simulink library "X8_lib"  (R2015a)
settings: Solver=ode45  StartTime=0.0  StopTime=10.0  RelTol=1e-3
values from neighbouring files (symbols this model uses):
  P = computeGains(T_phi_delta_a,T_v_delta_r,T_theta_delta_e,T_Va_theta,T_Va_delta_t,P)    [initX8_demo.m]
  T_elevon2ailelev = [1 1 ... (first row only)    [init.m]
  x0 = [eta_0', ny_0' zeros(1,6)]'    [init.m]    (also in runX8.m = [-0.0000    0.0000 -100.0000   0.9997    0.0000    0.0232   ; trimX8.m = [0 0 -h_ini         quat0(1) quat0(2) quat0(3)   quat0(4)   )
undefined symbols (not defined in the file or in its folder): F, Light, MIL
libraries: aerolibactuator x6, aerolibutil x2, aerolibwind2 x2, aerolibtransform2 x1
settings Model: Creator=krisgry  LastModifiedBy=krisgry

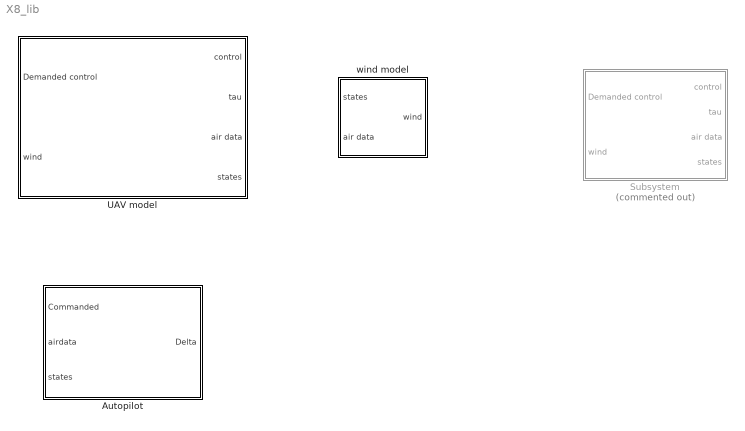
== system X8_lib ==
  Autopilot : Subsystem  mask{param='x8_param', X_trim=[0.0000    0.0000 -150.0000    0.9997    0.0000    0.0232   -0.0000 18.0168    0.0001    0.8366    0.0000    0.0000    0.0000 0.0039 -0.0000    0.0039   -0.0000    0.1240]', U_trim=[0.0079    0.0000         0    0.1240]'}
      mask prompts: param "UAV model"
      mask help:
      | UAV model can be either 'x8_param' or 'aerosonde'
      |
      | # Inputs:
      | Commanded: a 3x1 vector consisting of desired [airspeed, height, course angle]
      | airdata: a 10-element bus with airspeed, alpha, beta ... see bus_definitions.m
      | states: a bus consisting of 6 buses: position, attitude, quaternion, velocity, angular velocity, acceleration. See bus_definitions.m
      |
      | # Outputs:
      | delta: the control vector calculated by the autopilot
      mask init:
      | if(~exist('P') || ~isfield(P,'course_ki'))
      |     init;
      |     P.tau = 1; %Time constant for the band-limited differentiator
      |     P.u_trim = U_trim;
      |     [T_phi_delta_a,T_chi_phi,T_theta_delta_e,T_h_theta,T_h_Va,T_Va_delta_t,T_Va_theta,T_v_delta_r]= compute_tf_model(X_trim,U_trim,P);
      |     P=computeGains(T_phi_delta_a,T_v_delta_r,T_theta_delta_e,T_Va_theta,T_Va_delta_t,P);
      |    [phi0,theta0,psi0] = q2euler(X_trim(4:7)/norm(X_trim(4:7))); 
      | end
  Subsystem : Subsystem  Commented=on  mask{param='x8_param', pos0=[0 0 0], quat0=[1,0,0,0], vel0=[0 0 0], rate0=[0,0,0], servoR_pos0=0, servoR_vel0=0, servoL_pos0=0, servoL_vel0=0, prop_speed0=0}
      mask prompts: param "UAV model"; pos0 "NED position"; quat0 "Quaternion"; vel0 "Velocity"; rate0 "Angular velocity"; servoR_pos0 "Right servo deflection"; servoR_vel0 "Right servo deflection"; servoL_pos0 "Left servo deflection"; servoL_vel0 "Left servo speed"; prop_speed0 "Motor speed"
      mask help:
      | UAV model can be either 'x8_param' or 'aerosonde'
      |
      | #### Inputs:
      | Demanded control: a 4x1 vector consisting of [elevator, aileron, rudder, throttle]
      | wind: a 6x1 vector consisting of the wind+gust in NED, and the body rate gusts: [N,E,D,p,q,r]
      |
      | #### Outputs:
      | control: the control vector after it has been passed through the actuator model
      | tau: a 6x1 force/moment vector: [Fx,Fy,Fz,l,m,n]
      | airdata: a 10-element bus with airspeed, alpha, beta ... see bus_definitions.m
      | states: a bus consisting of 6 buses: position, attitude, quaternion, velocity, angular velocity, acceleration. See bus_definitions.m
      mask init:
      | % if(~exist('States') || ~isfield(States,'Quaternion'))
      | %     bus_defintions;
      | % end
      | x0 = [pos0,quat0,vel0,rate0,servoR_pos0,servoR_vel0,servoL_pos0,servoL_vel0,prop_speed0]
      | if(~exist('P') || ~isfield(P,'b'))
      |     init;
      | end
      mask DialogControl Container6 Prompt: Initial conditions
  UAV model : Subsystem  mask{param='x8_param', pos0=[0,0,0], quat0=[1,0,0,0], vel0=[0,0,0], rate0=[0,0,0], servoR_pos0=0, servoR_vel0=0, servoL_pos0=0, servoL_vel0=0, motor_speed0=0}
      mask prompts: param "UAV model"; pos0 "NED Position"; quat0 "Quaternion"; vel0 "Velocity"; rate0 "Angular Velocity"; servoR_pos0 "Right servo deflection"; servoR_vel0 "Right servo velocity"; servoL_pos0 "Left servo deflection"; servoL_vel0 "Left servo velocity"; motor_speed0 "Motor speed"
      mask help:
      | UAV model can be either 'x8_param' or 'aerosonde'
      |
      | # Inputs:
      | Demanded control: a 4x1 vector consisting of [elevator, aileron, rudder, throttle]
      | wind: a 6x1 vector consisting of the wind+gust in NED, and the body rate gusts: [N,E,D,p,q,r]
      |
      | # Outputs:
      | control: the control vector after it has been passed through the actuator model
      | tau: a 6x1 force/moment vector: [Fx,Fy,Fz,l,m,n]
      | airdata: a 10-element bus with airspeed, alpha, beta ... see bus_definitions.m
      | states: a bus consisting of 6 buses: position, attitude, quaternion, velocity, angular velocity, acceleration. See bus_definitions.m
      mask init:
      | %bus_defintions;
      | if(~exist('P') || ~isfield(P,'b'))
      |     init;
      | end
      mask DialogControl Container3 Prompt: Initial conditions
      mask Display:
      | image('X8.png')
      | port_label('output',1,'\delta','texmode','on')
      | port_label('output',2,'\tau','texmode','on')
      | port_label('output',3,'AirData','texmode','on')
      | port_label('output',4,'States','texmode','on')
      | port_label('input',1,'\delta_{demand}','texmode','on')
      | port_label('input',2,'Wind','texmode','on')
  wind model : Subsystem  mask{wind_speed=0, wind_dir=0, wind_start_time=0, param='x8_param'}
      mask prompts: wind_speed "Wind speed"; wind_dir "Wind direction"; wind_start_time "Wind start time"; param "UAV model"
      mask help: UAV model can be either 'x8_param' or 'aerosonde'
      mask init:
      | if(~exist('P') || ~isfield(P,'b'))
      |     init;
      | end

== system X8_lib/Autopilot ==
  Commanded : Inport
  airdata : Inport  Port=2
  states : Inport  Port=3
  Delay2 : Delay  DelayLength=1  InitialCondition=|  InputProcessing=Inherited  SampleTime=P.Ts
      | struct('Position',struct(...
      |                     'p_N', X_trim(1),...
      |                     'p_E', X_trim(2),...
      |                     'p_D', X_trim(3)),...
      |         'Attitude',struct(...
      |                     'phi', phi0,...
      |                     'theta', theta0,...
      |                     'psi', psi0),...
      |         'Quaternion',struct(...
      |                      'ScalarPart', X_trim(4),...
      |                     'VectorPart', [X_trim(5),X_trim(6),X_trim(7)]),...
      |         'Velocity',struct(...
      |                      'u', X_trim(8),...
      |                     'v', X_trim(9),...
      |                     'w', X_trim(10)),...
      |         'AngularVelocity', struct(...
      |                     'p', X_trim(11),...
      |                     'q', X_trim(12),...
      |                     'r', X_trim(13)),...
      |         'Acceleration', struct(...
      |                     'a_x', 0,...
      |                     'a_y', 0,...
      |                     'a_z', 0));
  Delay3 : Delay  DelayLength=1  InitialCondition=|  InputProcessing=Inherited  SampleTime=P.Ts
      | struct('Va', norm(X_trim(8:10)),...
      |         'alpha', 0,...
      |         'beta', 0,...
      |         'Course_angle', 0,...
      |         'Crab_angle', 0,...
      |         'Path_angle', 0,...
      |         'Air_mass_referenced_path_angle', 0,...
      |         'wind_x', 0,...
      |         'wind_y', 0,...
      |         'wind_z', 0);
  MATLAB Function : MATLAB Function  TreatAsAtomicUnit=on
  To Workspace3 : ToWorkspace  VariableName=delta1  SaveFormat=Structure With Time  SampleTime=-1
  Delta : Outport
  wires:
  Commanded/1 -> MATLAB Function/2(command)
  airdata/1 -> Delay3/1
  states/1 -> Delay2/1
  Delay3/1 -> MATLAB Function/3(airdata)
  Delay2/1 -> MATLAB Function/1(states)
  MATLAB Function/1(delta) -> Delta/1, To Workspace3/1

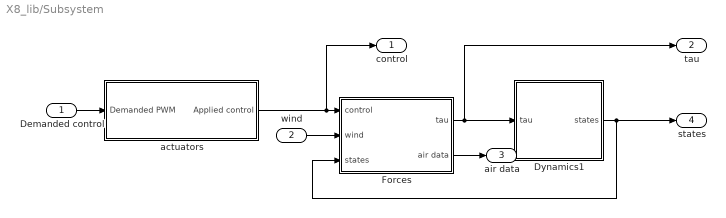
== system X8_lib/Subsystem ==
  Demanded control : Inport
  wind : Inport  Port=2  PortDimensions=6
  Dynamics1 : Subsystem
  Forces : Subsystem
  actuators : Subsystem
  control : Outport
  tau : Outport  Port=2
  air data : Outport  Port=3  OutDataTypeStr=Bus: AirData
  states : Outport  Port=4  OutDataTypeStr=Bus: States
  wires:
  Demanded control/1 -> actuators/1(Demanded PWM)
  actuators/1(Applied control) -> control/1, Forces/1(control)
  Forces/1(tau) -> tau/1, Dynamics1/1(tau)
  Forces/2(air data) -> air data/1
  Dynamics1/1(states) -> states/1, Forces/3(states)
  wind/1 -> Forces/2(wind)

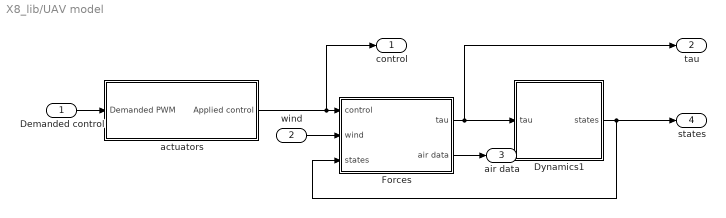
== system X8_lib/UAV model ==
  Demanded control : Inport
  wind : Inport  Port=2  PortDimensions=6
  Dynamics1 : Subsystem
  Forces : Subsystem
  actuators : Subsystem
  control : Outport
  tau : Outport  Port=2
  air data : Outport  Port=3  OutDataTypeStr=Bus: AirData
  states : Outport  Port=4  OutDataTypeStr=Bus: States
  wires:
  wind/1 -> Forces/2(wind)
  Demanded control/1 -> actuators/1(Demanded PWM)
  Forces/1(tau) -> tau/1, Dynamics1/1(tau)
  Dynamics1/1(states) -> states/1, Forces/3(states)
  Forces/2(air data) -> air data/1
  actuators/1(Applied control) -> control/1, Forces/1(control)

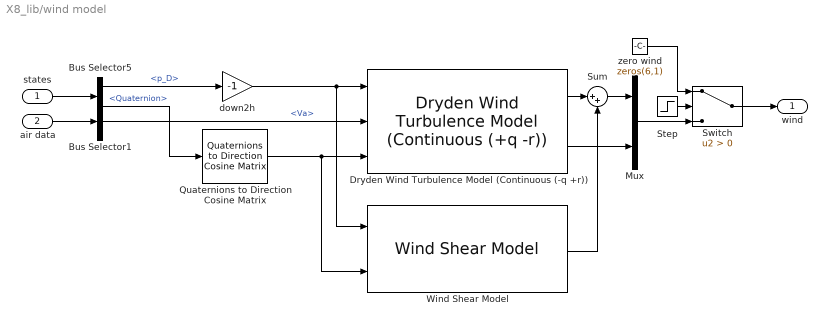
== system X8_lib/wind model ==
  states : Inport
  air data : Inport  Port=2
  Bus Selector1 : BusSelector  OutputSignals=Va
  Bus Selector5 : BusSelector  OutputSignals=Position.p_D,Quaternion
  Dryden Wind Turbulence Model (Continuous (-q +r)) : aerolibwind2/Dryden Wind Turbulence Model  (Continuous (+q -r))  units=Metric (MKS)  spec=MIL-F-8785C  model=Continuous Dryden (-q +r)  W20=wind_speed  Wdeg=wind_dir  TurbProb=10^-2 - Light  L_high=533.4  Wingspan=P.b  ts=0.1  Seed=[23341 23342 23343 23344]  T_on=on
  Mux : Mux  Inputs=2
  Quaternions to Direction Cosine Matrix : aerolibtransform2/Quaternions to  Direction Cosine Matrix
  Step : Step  Time=wind_start_time  Before=1  After=0  SampleTime=0
  Sum : Sum  Inputs=|++
  Switch : Switch  Criteria=u2 > Threshold
  Wind Shear Model : aerolibwind2/Wind Shear Model  units=Metric (MKS)  phase=Category C - Terminal Flight Phase  W_20=wind_speed  Wdeg=wind_dir
  down2h : Gain  Gain=-1
  zero wind : Constant  Value=zeros(6,1)
  wind : Outport
  wires:
  Bus Selector5/1 -> down2h/1  "<p_D>"
  Quaternions to Direction Cosine Matrix/1 -> Wind Shear Model/2, Dryden Wind Turbulence Model (Continuous (-q +r))/3
  Bus Selector1/1 -> Dryden Wind Turbulence Model (Continuous (-q +r))/2  "<Va>"
  Dryden Wind Turbulence Model (Continuous (-q +r))/2 -> Mux/2
  zero wind/1 -> Switch/1
  Switch/1 -> wind/1
  Bus Selector5/2 -> Quaternions to Direction Cosine Matrix/1  "<Quaternion>"
  air data/1 -> Bus Selector1/1
  states/1 -> Bus Selector5/1
  down2h/1 -> Wind Shear Model/1, Dryden Wind Turbulence Model (Continuous (-q +r))/1
  Step/1 -> Switch/2
  Mux/1 -> Switch/3
  Dryden Wind Turbulence Model (Continuous (-q +r))/1 -> Sum/1
  Sum/1 -> Mux/1
  Wind Shear Model/1 -> Sum/2

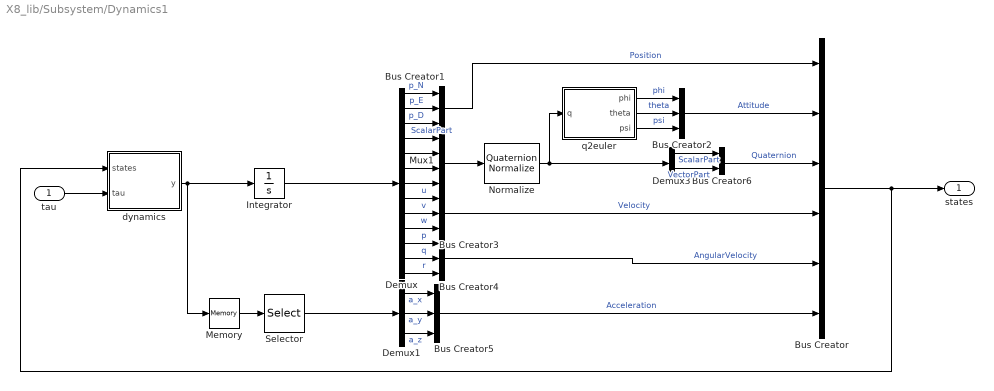
== system X8_lib/Subsystem/Dynamics1 ==
  tau : Inport
  Bus Creator : BusCreator  Inputs=6  OutDataTypeStr=Bus: States
  Bus Creator1 : BusCreator  Inputs=3  OutDataTypeStr=Bus: Position
  Bus Creator2 : BusCreator  Inputs=3  OutDataTypeStr=Bus: Attitude
  Bus Creator3 : BusCreator  Inputs=3  OutDataTypeStr=Bus: Velocity
  Bus Creator4 : BusCreator  Inputs=3  OutDataTypeStr=Bus: AngularVelocity
  Bus Creator5 : BusCreator  Inputs=3  OutDataTypeStr=Bus: Acceleration
  Bus Creator6 : BusCreator  Inputs=2  OutDataTypeStr=Bus: Quaternion
  Demux : Demux  Outputs=13
  Demux1 : Demux  Outputs=3
  Demux3 : Demux  Outputs=[1,3]
  Integrator : Integrator  InitialCondition=x0(1:13)
  Memory : Memory
  Mux1 : Mux
  Normalize : aerolibutil/Quaternion Normalize
  Selector : Selector  InputPortWidth=13  Indices=8:10
  dynamics : MATLAB Function  TreatAsAtomicUnit=on
  q2euler : MATLAB Function  TreatAsAtomicUnit=on
  states : Outport
  wires:
  dynamics/1(y) -> Memory/1, Integrator/1
  tau/1 -> dynamics/2(tau)
  Bus Creator/1 -> states/1, dynamics/1(states)
  Demux/2 -> Bus Creator1/2  "p_E"
  Demux/3 -> Bus Creator1/3  "p_D"
  Demux/1 -> Bus Creator1/1  "p_N"
  q2euler/2(theta) -> Bus Creator2/2  "theta"
  q2euler/3(psi) -> Bus Creator2/3  "psi"
  q2euler/1(phi) -> Bus Creator2/1  "phi"
  Demux/10 -> Bus Creator3/3  "w"
  Demux/8 -> Bus Creator3/1  "u"
  Demux/9 -> Bus Creator3/2  "v"
  Demux/11 -> Bus Creator4/1  "p"
  Demux/13 -> Bus Creator4/3  "r"
  Demux/12 -> Bus Creator4/2  "q"
  Bus Creator3/1 -> Bus Creator/4  "Velocity"
  Bus Creator1/1 -> Bus Creator/1  "Position"
  Bus Creator4/1 -> Bus Creator/5  "AngularVelocity"
  Bus Creator5/1 -> Bus Creator/6  "Acceleration"
  Selector/1 -> Demux1/1
  Demux1/1 -> Bus Creator5/1  "a_x"
  Demux1/2 -> Bus Creator5/2  "a_y"
  Demux1/3 -> Bus Creator5/3  "a_z"
  Demux/6 -> Mux1/3
  Demux/7 -> Mux1/4
  Demux/5 -> Mux1/2
  Normalize/1 -> q2euler/1(q), Demux3/1
  Integrator/1 -> Demux/1
  Demux3/1 -> Bus Creator6/1  "ScalarPart"
  Demux3/2 -> Bus Creator6/2  "VectorPart"
  Bus Creator6/1 -> Bus Creator/3  "Quaternion"
  Demux/4 -> Mux1/1  "ScalarPart"
  Bus Creator2/1 -> Bus Creator/2  "Attitude"
  Mux1/1 -> Normalize/1
  Memory/1 -> Selector/1

== system X8_lib/Subsystem/Forces ==
  control : Inport
  wind : Inport  Port=2
  states : Inport  Port=3
  MATLAB Function : MATLAB Function  TreatAsAtomicUnit=on
  Memory : Memory  X0=1e-15
  tau : Outport
  air data : Outport  Port=2
  tag scope: prop_torque=global, tau=global
  wires:
  states/1 -> MATLAB Function/1(states)
  control/1 -> MATLAB Function/3(control)
  wind/1 -> MATLAB Function/2(wind)
  MATLAB Function/1(tau) -> [tau], tau/1
  MATLAB Function/3(prop_torque) -> [prop_torque]
  Memory/1 -> air data/1
  MATLAB Function/2(AirData) -> Memory/1

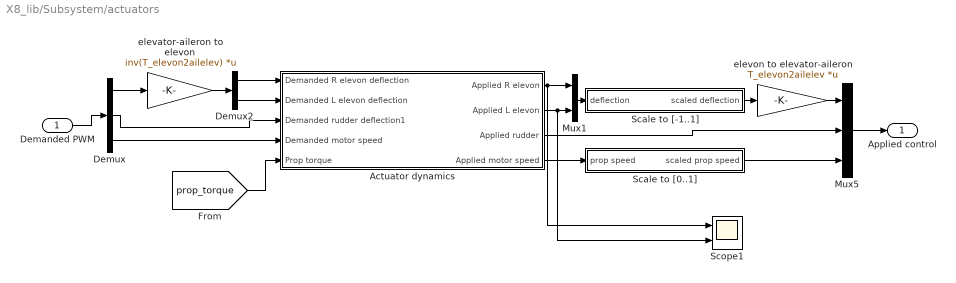
== system X8_lib/Subsystem/actuators ==
  Demanded PWM : Inport
  Actuator dynamics : Subsystem
  Demux : Demux  Outputs=[2,1,1]
  Demux2 : Demux  Outputs=2
  Mux1 : Mux  Inputs=2
  Mux5 : Mux  Inputs=3
  Scale to [-1..1] : Subsystem
  Scale to [0..1] : Subsystem
  Scope1 : Scope  NumInputPorts=2
      settings: YMin=-0.110121~-5  YMax=-0.0996332~5  SaveName=ScopeData23
  elevator-aileron to elevon : Gain  Gain=inv(T_elevon2ailelev)  Multiplication=Matrix(K*u) (u vector)
  elevon to elevator-aileron : Gain  Gain=T_elevon2ailelev  Multiplication=Matrix(K*u) (u vector)
  Applied control : Outport
  wires:
  Demanded PWM/1 -> Demux/1
  Demux2/2 -> Actuator dynamics/2("Demanded L elevon deflection ")
  elevator-aileron to elevon/1 -> Demux2/1
  Demux/1 -> elevator-aileron to elevon/1
  Demux2/1 -> Actuator dynamics/1(Demanded R elevon deflection)
  Actuator dynamics/2(Applied L elevon) -> Scope1/2, Mux1/2
  Actuator dynamics/4(Applied motor speed) -> Scale to [0..1]/1(prop speed)
  Scale to [-1..1]/1(scaled deflection) -> elevon to elevator-aileron/1
  elevon to elevator-aileron/1 -> Mux5/1
  Actuator dynamics/3(Applied rudder) -> Mux5/2
  Scale to [0..1]/1(scaled prop speed) -> Mux5/3
  Actuator dynamics/1(Applied R elevon) -> Scope1/1, Mux1/1
  Mux1/1 -> Scale to [-1..1]/1(deflection)
  Demux/2 -> Actuator dynamics/3(Demanded rudder deflection1)
  Mux5/1 -> Applied control/1
  [prop_torque] -> Actuator dynamics/5(Prop torque)
  Demux/3 -> Actuator dynamics/4(Demanded motor speed)

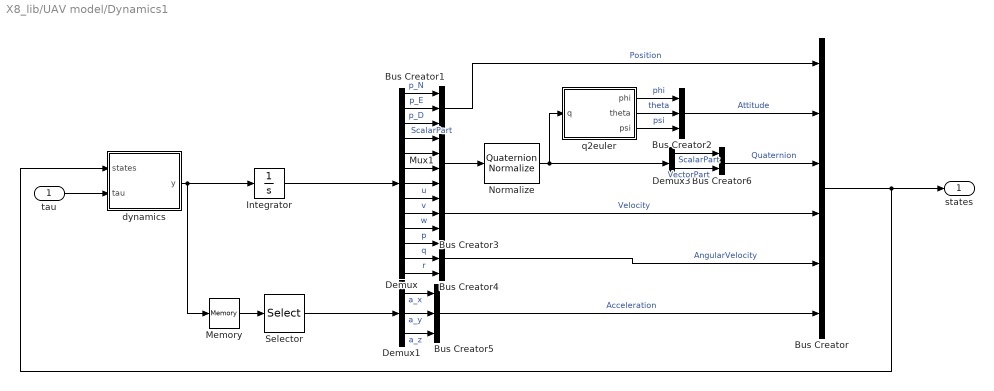
== system X8_lib/UAV model/Dynamics1 ==
  tau : Inport
  Bus Creator : BusCreator  Inputs=6  OutDataTypeStr=Bus: States
  Bus Creator1 : BusCreator  Inputs=3  OutDataTypeStr=Bus: Position
  Bus Creator2 : BusCreator  Inputs=3  OutDataTypeStr=Bus: Attitude
  Bus Creator3 : BusCreator  Inputs=3  OutDataTypeStr=Bus: Velocity
  Bus Creator4 : BusCreator  Inputs=3  OutDataTypeStr=Bus: AngularVelocity
  Bus Creator5 : BusCreator  Inputs=3  OutDataTypeStr=Bus: Acceleration
  Bus Creator6 : BusCreator  Inputs=2  OutDataTypeStr=Bus: Quaternion
  Demux : Demux  Outputs=13
  Demux1 : Demux  Outputs=3
  Demux3 : Demux  Outputs=[1,3]
  Integrator : Integrator  InitialCondition=[pos0,quat0,vel0,rate0]%x0(1:13)
  Memory : Memory
  Mux1 : Mux
  Normalize : aerolibutil/Quaternion Normalize
  Selector : Selector  InputPortWidth=13  Indices=8:10
  dynamics : MATLAB Function  TreatAsAtomicUnit=on
  q2euler : MATLAB Function  TreatAsAtomicUnit=on
  states : Outport
  wires:
  dynamics/1(y) -> Memory/1, Integrator/1
  tau/1 -> dynamics/2(tau)
  Bus Creator/1 -> states/1, dynamics/1(states)
  Demux/2 -> Bus Creator1/2  "p_E"
  Demux/3 -> Bus Creator1/3  "p_D"
  Demux/1 -> Bus Creator1/1  "p_N"
  q2euler/2(theta) -> Bus Creator2/2  "theta"
  q2euler/3(psi) -> Bus Creator2/3  "psi"
  q2euler/1(phi) -> Bus Creator2/1  "phi"
  Demux/10 -> Bus Creator3/3  "w"
  Demux/8 -> Bus Creator3/1  "u"
  Demux/9 -> Bus Creator3/2  "v"
  Demux/11 -> Bus Creator4/1  "p"
  Demux/13 -> Bus Creator4/3  "r"
  Demux/12 -> Bus Creator4/2  "q"
  Bus Creator3/1 -> Bus Creator/4  "Velocity"
  Bus Creator1/1 -> Bus Creator/1  "Position"
  Bus Creator4/1 -> Bus Creator/5  "AngularVelocity"
  Bus Creator5/1 -> Bus Creator/6  "Acceleration"
  Selector/1 -> Demux1/1
  Demux1/1 -> Bus Creator5/1  "a_x"
  Demux1/2 -> Bus Creator5/2  "a_y"
  Demux1/3 -> Bus Creator5/3  "a_z"
  Demux/6 -> Mux1/3
  Demux/7 -> Mux1/4
  Demux/5 -> Mux1/2
  Normalize/1 -> q2euler/1(q), Demux3/1
  Integrator/1 -> Demux/1
  Demux3/1 -> Bus Creator6/1  "ScalarPart"
  Demux3/2 -> Bus Creator6/2  "VectorPart"
  Bus Creator6/1 -> Bus Creator/3  "Quaternion"
  Demux/4 -> Mux1/1  "ScalarPart"
  Bus Creator2/1 -> Bus Creator/2  "Attitude"
  Mux1/1 -> Normalize/1
  Memory/1 -> Selector/1

== system X8_lib/UAV model/Forces ==
  control : Inport
  wind : Inport  Port=2
  states : Inport  Port=3
  Goto1 : Goto  Commented=on  GotoTag=tau  TagVisibility=global
  MATLAB Function : MATLAB Function  TreatAsAtomicUnit=on
  Memory : Memory  X0=1e-15
  tau : Outport
  air data : Outport  Port=2
  tag scope: prop_torque=global
  wires:
  states/1 -> MATLAB Function/1(states)
  control/1 -> MATLAB Function/3(control)
  wind/1 -> MATLAB Function/2(wind)
  MATLAB Function/1(tau) -> Goto1/1, tau/1
  MATLAB Function/3(prop_torque) -> [prop_torque]
  Memory/1 -> air data/1
  MATLAB Function/2(AirData) -> Memory/1

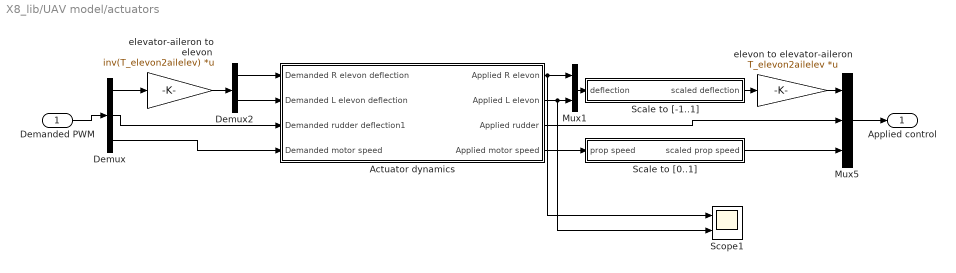
== system X8_lib/UAV model/actuators ==
  Demanded PWM : Inport
  Actuator dynamics : Subsystem
  Demux : Demux  Outputs=[2,1,1]
  Demux2 : Demux  Outputs=2
  Mux1 : Mux  Inputs=2
  Mux5 : Mux  Inputs=3
  Scale to [-1..1] : Subsystem
  Scale to [0..1] : Subsystem
  Scope1 : Scope  NumInputPorts=2
      settings: YMin=-0.110121~-5  YMax=-0.0996332~5  SaveName=ScopeData23
  elevator-aileron to elevon : Gain  Gain=inv(T_elevon2ailelev)  Multiplication=Matrix(K*u) (u vector)
  elevon to elevator-aileron : Gain  Gain=T_elevon2ailelev  Multiplication=Matrix(K*u) (u vector)
  Applied control : Outport
  wires:
  Demanded PWM/1 -> Demux/1
  Demux2/2 -> Actuator dynamics/2("Demanded L elevon deflection ")
  elevator-aileron to elevon/1 -> Demux2/1
  Demux/1 -> elevator-aileron to elevon/1
  Demux2/1 -> Actuator dynamics/1(Demanded R elevon deflection)
  Actuator dynamics/2(Applied L elevon) -> Scope1/2, Mux1/2
  Actuator dynamics/4(Applied motor speed) -> Scale to [0..1]/1(prop speed)
  Scale to [-1..1]/1(scaled deflection) -> elevon to elevator-aileron/1
  elevon to elevator-aileron/1 -> Mux5/1
  Actuator dynamics/3(Applied rudder) -> Mux5/2
  Scale to [0..1]/1(scaled prop speed) -> Mux5/3
  Actuator dynamics/1(Applied R elevon) -> Scope1/1, Mux1/1
  Mux1/1 -> Scale to [-1..1]/1(deflection)
  Demux/2 -> Actuator dynamics/3(Demanded rudder deflection1)
  Mux5/1 -> Applied control/1
  Demux/3 -> Actuator dynamics/4(Demanded motor speed)

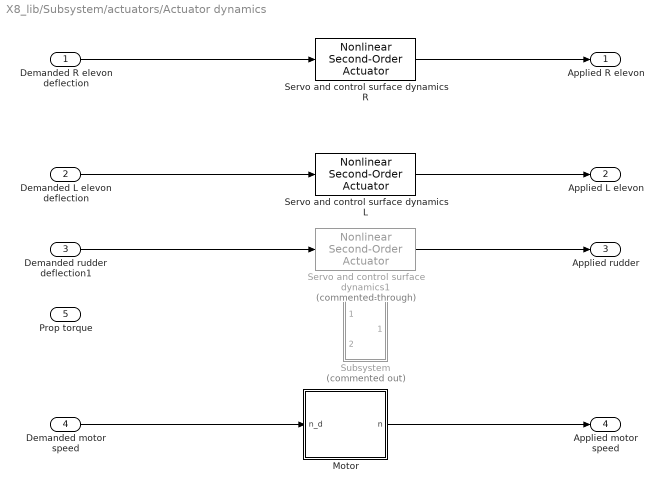
== system X8_lib/Subsystem/actuators/Actuator dynamics ==
  Demanded R elevon deflection : Inport
  "Demanded L elevon deflection " : Inport  Port=2
  Demanded rudder deflection1 : Inport  Port=3
  Demanded motor speed : Inport  Port=4
  Prop torque : Inport  Port=5
  Motor : Subsystem  mask{T=0.2, X0=x0(18)}
      mask prompts: T "Time constant"; X0 "Initial condition"
      mask DialogControl DescTextVar Prompt: Simple first order motor model
  Servo and control surface dynamics L : aerolibactuator/Nonlinear Second-Order Actuator  wn_fin=P.servo.omega0  z_fin=P.servo.zeta  fin_max=P.servo.max_rad  fin_min=P.servo.min_rad  fin_maxrate=P.servo.rate_lim  fin_act_0=x0(16)  fin_act_vel=x0(17)
  Servo and control surface dynamics R : aerolibactuator/Nonlinear Second-Order Actuator  wn_fin=P.servo.omega0  z_fin=P.servo.zeta  fin_max=P.servo.max_rad  fin_min=P.servo.min_rad  fin_maxrate=P.servo.rate_lim  fin_act_0=x0(14)  fin_act_vel=x0(15)
  Servo and control surface dynamics1 : aerolibactuator/Nonlinear Second-Order Actuator  Commented=through  wn_fin=P.servo.omega0  z_fin=P.servo.zeta  fin_max=P.servo.max_rad  fin_min=P.servo.min_rad  fin_maxrate=P.servo.rate_lim  fin_act_0=P.servo.pos0  fin_act_vel=P.servo.rate0
  Subsystem : Subsystem  Commented=on
  Applied R elevon : Outport
  Applied L elevon : Outport  Port=2
  Applied rudder : Outport  Port=3
  Applied motor speed : Outport  Port=4
  wires:
  Servo and control surface dynamics R/1 -> Applied R elevon/1
  Motor/1(n) -> Applied motor speed/1
  Servo and control surface dynamics1/1 -> Applied rudder/1
  Servo and control surface dynamics L/1 -> Applied L elevon/1
  Demanded R elevon deflection/1 -> Servo and control surface dynamics R/1
  "Demanded L elevon deflection "/1 -> Servo and control surface dynamics L/1
  Demanded rudder deflection1/1 -> Servo and control surface dynamics1/1
  Demanded motor speed/1 -> Motor/1(n_d)

== system X8_lib/Subsystem/actuators/Scale to [-1..1] ==
  deflection : Inport
  Gain : Gain  Gain=P.rad2unit
  Saturation : Saturate  UpperLimit=1  LowerLimit=-1
  scaled deflection : Outport
  wires:
  deflection/1 -> Gain/1
  Gain/1 -> Saturation/1
  Saturation/1 -> scaled deflection/1

== system X8_lib/Subsystem/actuators/Scale to [0..1] ==
  prop speed : Inport
  Gain : Gain  Commented=through  Gain=1/P.motor.omega_max
  Saturation : Saturate  UpperLimit=1  LowerLimit=0
  scaled prop speed : Outport
  wires:
  prop speed/1 -> Gain/1
  Gain/1 -> Saturation/1
  Saturation/1 -> scaled prop speed/1

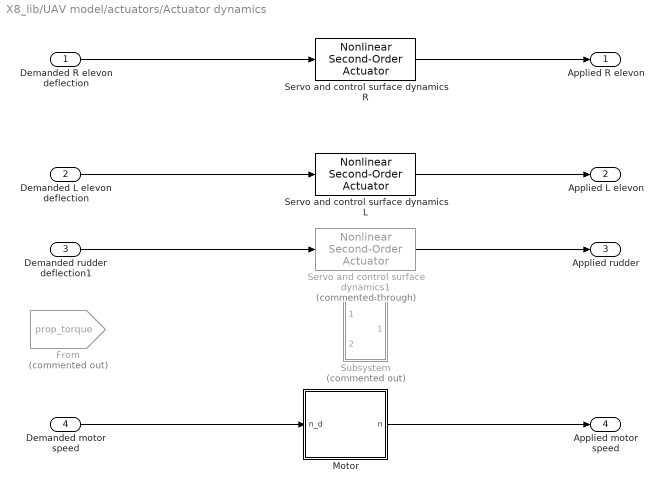
== system X8_lib/UAV model/actuators/Actuator dynamics ==
  Demanded R elevon deflection : Inport
  "Demanded L elevon deflection " : Inport  Port=2
  Demanded rudder deflection1 : Inport  Port=3
  Demanded motor speed : Inport  Port=4
  From : From  Commented=on  GotoTag=prop_torque  TagVisibility=global
  Motor : Subsystem  mask{T=0.2, X0=motor_speed0}
      mask prompts: T "Time constant"; X0 "Initial condition"
      mask DialogControl DescTextVar Prompt: Simple first order motor model
  Servo and control surface dynamics L : aerolibactuator/Nonlinear Second-Order Actuator  wn_fin=P.servo.omega0  z_fin=P.servo.zeta  fin_max=P.servo.max_rad  fin_min=P.servo.min_rad  fin_maxrate=P.servo.rate_lim  fin_act_0=servoL_pos0  fin_act_vel=servoL_vel0
  Servo and control surface dynamics R : aerolibactuator/Nonlinear Second-Order Actuator  wn_fin=P.servo.omega0  z_fin=P.servo.zeta  fin_max=P.servo.max_rad  fin_min=P.servo.min_rad  fin_maxrate=P.servo.rate_lim  fin_act_0=servoR_pos0  fin_act_vel=servoR_vel0
  Servo and control surface dynamics1 : aerolibactuator/Nonlinear Second-Order Actuator  Commented=through  wn_fin=P.servo.omega0  z_fin=P.servo.zeta  fin_max=P.servo.max_rad  fin_min=P.servo.min_rad  fin_maxrate=P.servo.rate_lim  fin_act_0=P.servo.pos0  fin_act_vel=P.servo.rate0
  Subsystem : Subsystem  Commented=on
  Applied R elevon : Outport
  Applied L elevon : Outport  Port=2
  Applied rudder : Outport  Port=3
  Applied motor speed : Outport  Port=4
  wires:
  Servo and control surface dynamics R/1 -> Applied R elevon/1
  Motor/1(n) -> Applied motor speed/1
  Servo and control surface dynamics1/1 -> Applied rudder/1
  Servo and control surface dynamics L/1 -> Applied L elevon/1
  Demanded R elevon deflection/1 -> Servo and control surface dynamics R/1
  "Demanded L elevon deflection "/1 -> Servo and control surface dynamics L/1
  Demanded rudder deflection1/1 -> Servo and control surface dynamics1/1
  Demanded motor speed/1 -> Motor/1(n_d)

== system X8_lib/UAV model/actuators/Scale to [-1..1] ==
  deflection : Inport
  Gain : Gain  Gain=P.rad2unit
  Saturation : Saturate  UpperLimit=1  LowerLimit=-1
  scaled deflection : Outport
  wires:
  deflection/1 -> Gain/1
  Gain/1 -> Saturation/1
  Saturation/1 -> scaled deflection/1

== system X8_lib/UAV model/actuators/Scale to [0..1] ==
  prop speed : Inport
  Gain : Gain  Commented=through  Gain=1/P.motor.omega_max
  Saturation : Saturate  UpperLimit=1  LowerLimit=0
  scaled prop speed : Outport
  wires:
  prop speed/1 -> Gain/1
  Gain/1 -> Saturation/1
  Saturation/1 -> scaled prop speed/1

== system X8_lib/Subsystem/actuators/Actuator dynamics/Motor ==
  n_d : Inport
  1/T : Gain  Gain=1/T
  Integrator : Integrator  InitialCondition=X0  ContinuousStateAttributes='throttle'
  Sum : Sum  Inputs=|+-
  n : Outport
  wires:
  Integrator/1 -> n/1, Sum/2
  n_d/1 -> Sum/1
  Sum/1 -> 1/T/1
  1/T/1 -> Integrator/1

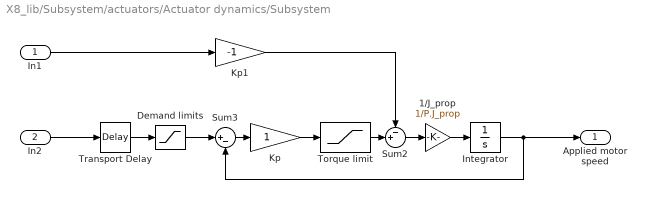
== system X8_lib/Subsystem/actuators/Actuator dynamics/Subsystem ==
  In1 : Inport
  In2 : Inport  Port=2
  1/J_prop : Gain  Gain=1/P.J_prop  SaturateOnIntegerOverflow=on  OutDataTypeStr=Inherit: Same as input  ParamDataTypeStr=Inherit: Same as input
  Demand limits : Saturate  UpperLimit=1  LowerLimit=0
  Integrator : Integrator  InitialCondition=0.5
  Kp : Gain  SaturateOnIntegerOverflow=on  OutDataTypeStr=Inherit: Same as input  ParamDataTypeStr=Inherit: Same as input
  Kp1 : Gain  Gain=-1  SaturateOnIntegerOverflow=on  OutDataTypeStr=Inherit: Same as input  ParamDataTypeStr=Inherit: Same as input
  Sum2 : Sum  Inputs=-+|  SaturateOnIntegerOverflow=on  InputSameDT=on  OutDataTypeStr=Inherit: Same as first input
  Sum3 : Sum  Inputs=|+-  SaturateOnIntegerOverflow=on  InputSameDT=on  OutDataTypeStr=Inherit: Same as first input
  Torque limit : Saturate  UpperLimit=P.motor.torque_max  LowerLimit=0  ZeroCross=off
  Transport Delay : TransportDelay  DelayTime=0.001  PadeOrder=1
  Applied motor speed : Outport
  wires:
  Demand limits/1 -> Sum3/1
  Sum3/1 -> Kp/1
  Integrator/1 -> Applied motor speed/1, Sum3/2
  Torque limit/1 -> Sum2/2
  Sum2/1 -> 1/J_prop/1
  1/J_prop/1 -> Integrator/1
  Kp/1 -> Torque limit/1
  In1/1 -> Kp1/1
  In2/1 -> Transport Delay/1
  Transport Delay/1 -> Demand limits/1
  Kp1/1 -> Sum2/1

== system X8_lib/UAV model/actuators/Actuator dynamics/Motor ==
  n_d : Inport
  1/T : Gain  Gain=1/T
  Integrator : Integrator  InitialCondition=X0  ContinuousStateAttributes='throttle'
  Sum : Sum  Inputs=|+-
  n : Outport
  wires:
  Integrator/1 -> n/1, Sum/2
  n_d/1 -> Sum/1
  Sum/1 -> 1/T/1
  1/T/1 -> Integrator/1

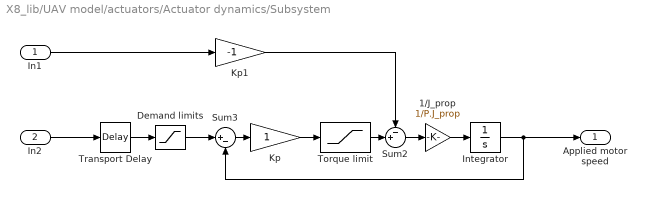
== system X8_lib/UAV model/actuators/Actuator dynamics/Subsystem ==
  In1 : Inport
  In2 : Inport  Port=2
  1/J_prop : Gain  Gain=1/P.J_prop  SaturateOnIntegerOverflow=on  OutDataTypeStr=Inherit: Same as input  ParamDataTypeStr=Inherit: Same as input
  Demand limits : Saturate  UpperLimit=1  LowerLimit=0
  Integrator : Integrator  InitialCondition=0.5
  Kp : Gain  SaturateOnIntegerOverflow=on  OutDataTypeStr=Inherit: Same as input  ParamDataTypeStr=Inherit: Same as input
  Kp1 : Gain  Gain=-1  SaturateOnIntegerOverflow=on  OutDataTypeStr=Inherit: Same as input  ParamDataTypeStr=Inherit: Same as input
  Sum2 : Sum  Inputs=-+|  SaturateOnIntegerOverflow=on  InputSameDT=on  OutDataTypeStr=Inherit: Same as first input
  Sum3 : Sum  Inputs=|+-  SaturateOnIntegerOverflow=on  InputSameDT=on  OutDataTypeStr=Inherit: Same as first input
  Torque limit : Saturate  UpperLimit=P.motor.torque_max  LowerLimit=0  ZeroCross=off
  Transport Delay : TransportDelay  DelayTime=0.001  PadeOrder=1
  Applied motor speed : Outport
  wires:
  Demand limits/1 -> Sum3/1
  Sum3/1 -> Kp/1
  Integrator/1 -> Applied motor speed/1, Sum3/2
  Torque limit/1 -> Sum2/2
  Sum2/1 -> 1/J_prop/1
  1/J_prop/1 -> Integrator/1
  Kp/1 -> Torque limit/1
  In1/1 -> Kp1/1
  In2/1 -> Transport Delay/1
  Transport Delay/1 -> Demand limits/1
  Kp1/1 -> Sum2/1

== matlab function X8_lib/UAV model/Forces/MATLAB Function ==
  data: states input; tau output; AirData output Bus: AirData; wind input; control input; P parameter; prop_torque output
function [tau,AirData,prop_torque]  = fcn(states,wind,control,P)
%#codegen
% ,Va, alpha, beta, course, crab, gamma, gamma_a, wind_b,T_prop
temp = forces([states.Position.p_N,states.Position.p_E,states.Position.p_D,states.Attitude.phi,states.Attitude.theta,states.Attitude.psi]',...
              [states.Velocity.u,states.Velocity.v,states.Velocity.w,states.AngularVelocity.p,states.AngularVelocity.q,states.AngularVelocity.r]',...
              [states.Quaternion.ScalarPart;states.Quaternion.VectorPart]',control,wind,P);
tau = temp(1:6);
AirData.Va                              = temp(7);
AirData.alpha                           = temp(8);
AirData.beta                            = temp(9);
AirData.Course_angle                    = temp(10);
AirData.Crab_angle                      = temp(11);
AirData.Path_angle                      = temp(12);
AirData.Air_mass_referenced_path_angle  = temp(13);
AirData.wind_x                          = temp(14);
AirData.wind_y                          = temp(15);
AirData.wind_z                          = temp(16);

prop_torque     = temp(17);

== matlab function X8_lib/UAV model/Dynamics1/q2euler ==
  data: q input; phi output; theta output; psi output
function [phi,theta,psi] = fcn(q)
%#codegen
[phi,theta,psi] = q2euler(q);
end

== matlab function X8_lib/UAV model/Dynamics1/dynamics ==
  data: states input Bus: States; tau input; y output; P parameter
function y = fcn(states,tau, P)
%#codegen

y = dynamics([states.Position.p_N,states.Position.p_E,states.Position.p_D]',[states.Quaternion.ScalarPart,states.Quaternion.VectorPart']',...
       [states.Velocity.u,states.Velocity.v,states.Velocity.w]',[states.AngularVelocity.p,states.AngularVelocity.q,states.AngularVelocity.r]',...
       tau,P);
% y = dynamics(states(1:3),states(4:7),states(8:10),states(11:13),tau,P);
end

== matlab function X8_lib/Subsystem/Dynamics1/dynamics ==
  data: states input Bus: States; tau input; y output; P parameter
function y = fcn(states,tau, P)
%#codegen

y = dynamics([states.Position.p_N,states.Position.p_E,states.Position.p_D]',[states.Quaternion.ScalarPart,states.Quaternion.VectorPart']',...
       [states.Velocity.u,states.Velocity.v,states.Velocity.w]',[states.AngularVelocity.p,states.AngularVelocity.q,states.AngularVelocity.r]',...
       tau,P);
% y = dynamics(states(1:3),states(4:7),states(8:10),states(11:13),tau,P);
end

== matlab function X8_lib/Subsystem/Dynamics1/q2euler ==
  data: q input; phi output; theta output; psi output
function [phi,theta,psi] = fcn(q)
%#codegen
[phi,theta,psi] = q2euler(q);
end

== matlab function X8_lib/Subsystem/Forces/MATLAB Function ==
  data: states input; tau output; AirData output Bus: AirData; wind input; control input; P parameter; prop_torque output
function [tau,AirData,prop_torque]  = fcn(states,wind,control,P)
%#codegen
% ,Va, alpha, beta, course, crab, gamma, gamma_a, wind_b,T_prop
temp = forces([states.Position.p_N,states.Position.p_E,states.Position.p_D,states.Attitude.phi,states.Attitude.theta,states.Attitude.psi]',...
              [states.Velocity.u,states.Velocity.v,states.Velocity.w,states.AngularVelocity.p,states.AngularVelocity.q,states.AngularVelocity.r]',...
              [states.Quaternion.ScalarPart;states.Quaternion.VectorPart]',control,wind,P);
tau = temp(1:6);
AirData.Va                              = temp(7);
AirData.alpha                           = temp(8);
AirData.beta                            = temp(9);
AirData.Course_angle                    = temp(10);
AirData.Crab_angle                      = temp(11);
AirData.Path_angle                      = temp(12);
AirData.Air_mass_referenced_path_angle  = temp(13);
AirData.wind_x                          = temp(14);
AirData.wind_y                          = temp(15);
AirData.wind_z                          = temp(16);

prop_torque     = temp(17);

== matlab function X8_lib/Autopilot/MATLAB Function ==
  data: states input; delta output; command input; airdata input; P parameter
function delta = fcn(states, command,airdata,P)
%#codegen

delta = autopilot([states.Position.p_N,states.Position.p_E,states.Position.p_D,states.Velocity.u,states.Velocity.v,states.Velocity.w,...
                    states.Attitude.phi,states.Attitude.theta,states.Attitude.psi,states.AngularVelocity.p,states.AngularVelocity.q,states.AngularVelocity.r,...
                    command',airdata.Va,airdata.alpha,airdata.beta,airdata.wind_x,airdata.wind_y,airdata.wind_z,airdata.Course_angle]',P);
end
